simulink model "scattering_based_bi_teleop_pp_kalman"  (R2020b)
settings: Solver=FixedStepAuto  StartTime=0.0  StopTime=30  FixedStep=Ts  RelTol=1e-3
values from neighbouring files (symbols this model uses):
  A = 1    [four_channel_bilateral_teleoperation_kalman_params.m]    (also in four_channel_bilateral_teleoperation_params.m; kalman_test.m = [1 Ts Ts^2/2; 0 1 Ts; 0 0 1]; recursive_estimation.m = [1 Ts Ts^2/2; 0 1 Ts; 0 0 1]; scattering_based_bi_teleop_pf_kalman_params.m)
  b = 1    [scattering_based_bi_teleop_pf_kalman_params.m]    (also in scattering_based_bi_teleop_pf_params.m; scattering_based_bi_teleop_pp_kalman_params.m; scattering_based_bi_teleop_pp_params.m; scattering_based_bilateral_teleoperation_pp_params.m = 0.234)
  Be = 100    [four_channel_bilateral_teleoperation_architecture_params.m]    (also in four_channel_bilateral_teleoperation_kalman_params.m = 0; four_channel_bilateral_teleoperation_params.m = 0; scattering_based_bi_teleop_pf_kalman_params.m = 10; scattering_based_bi_teleop_pf_params.m = 10)
  Bh = 70    [four_channel_bilateral_teleoperation_architecture_params.m]    (also in four_channel_bilateral_teleoperation_kalman_params.m; four_channel_bilateral_teleoperation_params.m = 1.5; scattering_based_bi_teleop_pf_kalman_params.m = 1.5; scattering_based_bi_teleop_pf_params.m = 1.5)
  Bm = 1    [four_channel_bilateral_teleoperation_architecture_params.m]    (also in four_channel_bilateral_teleoperation_kalman_params.m = 0.8; four_channel_bilateral_teleoperation_params.m = 0.8; scattering_based_bi_teleop_pf_kalman_params.m = 0; scattering_based_bi_teleop_pf_params.m = 0)
  Bs = 1    [four_channel_bilateral_teleoperation_architecture_params.m]    (also in four_channel_bilateral_teleoperation_kalman_params.m = 3.2; four_channel_bilateral_teleoperation_params.m = 3.2; scattering_based_bi_teleop_pf_kalman_params.m = 40; scattering_based_bi_teleop_pf_params.m = 80)
  delay = 10    [scattering_based_bi_teleop_pf_kalman_params.m]    (also in scattering_based_bi_teleop_pf_params.m; scattering_based_bi_teleop_pp_kalman_params.m = 2; scattering_based_bi_teleop_pp_params.m; tank_based_bi_teleop_pf_kalman.m = 1)
  Dm = 5    [four_channel_bilateral_teleoperation_architecture_params.m]    (also in four_channel_bilateral_teleoperation_kalman_params.m = 0; four_channel_bilateral_teleoperation_params.m = 0; scattering_based_bi_teleop_pf_kalman_params.m = 0; scattering_based_bi_teleop_pf_params.m = 0)
  Ds = 10    [four_channel_bilateral_teleoperation_architecture_params.m]    (also in four_channel_bilateral_teleoperation_kalman_params.m = 0; four_channel_bilateral_teleoperation_params.m = 0; scattering_based_bi_teleop_pf_kalman_params.m = 0; scattering_based_bi_teleop_pf_params.m = 0)
  Fc = 1    [four_channel_bilateral_teleoperation_kalman_params.m]    (also in four_channel_bilateral_teleoperation_params.m = 0.5; scattering_based_bi_teleop_pf_kalman_params.m = 0.1; scattering_based_bi_teleop_pf_params.m = 0.1; scattering_based_bi_teleop_pp_kalman_params.m = 0.1)
  Filter = 8    [scattering_based_bi_teleop_pf_kalman_params.m]    (also in scattering_based_bi_teleop_pf_params.m = 10; scattering_based_bi_teleop_pp_kalman_params.m = 10; scattering_based_bi_teleop_pp_params.m = 10; tank_based_bi_teleop_pf_kalman.m = 100)
  Fip = 1    [four_channel_bilateral_teleoperation_kalman_params.m]    (also in four_channel_bilateral_teleoperation_params.m; scattering_based_bi_teleop_pf_kalman_params.m = 5; scattering_based_bi_teleop_pf_params.m = 5; scattering_based_bi_teleop_pp_kalman_params.m = 5)
  Ih = 2    [scattering_based_bi_teleop_pf_kalman_params.m]    (also in scattering_based_bi_teleop_pf_params.m; scattering_based_bi_teleop_pp_kalman_params.m; scattering_based_bi_teleop_pp_params.m; tank_based_bi_teleop_pf_kalman.m)
  Je = 0    [four_channel_bilateral_teleoperation_architecture_params.m]    (also in four_channel_bilateral_teleoperation_kalman_params.m; four_channel_bilateral_teleoperation_params.m; scattering_based_bi_teleop_pf_kalman_params.m; scattering_based_bi_teleop_pf_params.m)
  Jh = 0.5    [four_channel_bilateral_teleoperation_architecture_params.m]    (also in four_channel_bilateral_teleoperation_kalman_params.m; four_channel_bilateral_teleoperation_params.m = 0; scattering_based_bi_teleop_pf_kalman_params.m = 0; scattering_based_bi_teleop_pf_params.m = 0)
  Ke = 200    [four_channel_bilateral_teleoperation_architecture_params.m]    (also in four_channel_bilateral_teleoperation_kalman_params.m = 50; four_channel_bilateral_teleoperation_params.m; scattering_based_bi_teleop_pf_kalman_params.m; scattering_based_bi_teleop_pf_params.m)
  Kh = 2000    [four_channel_bilateral_teleoperation_architecture_params.m]    (also in four_channel_bilateral_teleoperation_kalman_params.m; four_channel_bilateral_teleoperation_params.m = 1; scattering_based_bi_teleop_pf_kalman_params.m = 1; scattering_based_bi_teleop_pf_params.m = 1)
  Km = 1    [four_channel_bilateral_teleoperation_architecture_params.m]    (also in four_channel_bilateral_teleoperation_kalman_params.m; four_channel_bilateral_teleoperation_params.m; scattering_based_bi_teleop_pf_kalman_params.m = 0; scattering_based_bi_teleop_pf_params.m = 0)
  Ks = 1    [four_channel_bilateral_teleoperation_architecture_params.m]    (also in four_channel_bilateral_teleoperation_kalman_params.m = 4; four_channel_bilateral_teleoperation_params.m = 4; scattering_based_bi_teleop_pf_kalman_params.m = 50; scattering_based_bi_teleop_pf_params.m = 100)
  Mm = 0.5    [four_channel_bilateral_teleoperation_architecture_params.m]    (also in four_channel_bilateral_teleoperation_kalman_params.m; four_channel_bilateral_teleoperation_params.m; scattering_based_bi_teleop_pf_kalman_params.m; scattering_based_bi_teleop_pf_params.m)
  Ms = 2    [four_channel_bilateral_teleoperation_architecture_params.m]    (also in four_channel_bilateral_teleoperation_kalman_params.m; four_channel_bilateral_teleoperation_params.m; scattering_based_bi_teleop_pf_kalman_params.m; scattering_based_bi_teleop_pf_params.m)
  Ph = 2000    [four_channel_bilateral_teleoperation_kalman_params.m]    (also in four_channel_bilateral_teleoperation_params.m = 50; scattering_based_bi_teleop_pf_kalman_params.m = 5; scattering_based_bi_teleop_pf_params.m = 5; scattering_based_bi_teleop_pp_kalman_params.m = 6)
  Ts = 0.001    [four_channel_bilateral_teleoperation_kalman_params.m]    (also in four_channel_bilateral_teleoperation_params.m; kalman_test.m; recursive_estimation.m; scattering_based_bi_teleop_pf_kalman_params.m)
  VarianceForces = 0.01    [four_channel_bilateral_teleoperation_kalman_params.m]    (also in four_channel_bilateral_teleoperation_params.m = 0; scattering_based_bi_teleop_pf_kalman_params.m; scattering_based_bi_teleop_pp_kalman_params.m; scattering_based_bi_teleop_pp_params.m)
  VarianceVelocities = 0.001    [four_channel_bilateral_teleoperation_kalman_params.m]    (also in four_channel_bilateral_teleoperation_params.m = 0; scattering_based_bi_teleop_pf_kalman_params.m = 1e-05; scattering_based_bi_teleop_pp_kalman_params.m = 1e-05; scattering_based_bi_teleop_pp_params.m = 1e-05)
undefined symbols (not defined in the file or in its folder): DiscIntNeverNeededParam
settings Model: Creator=anuj  LastModifiedBy=filippo

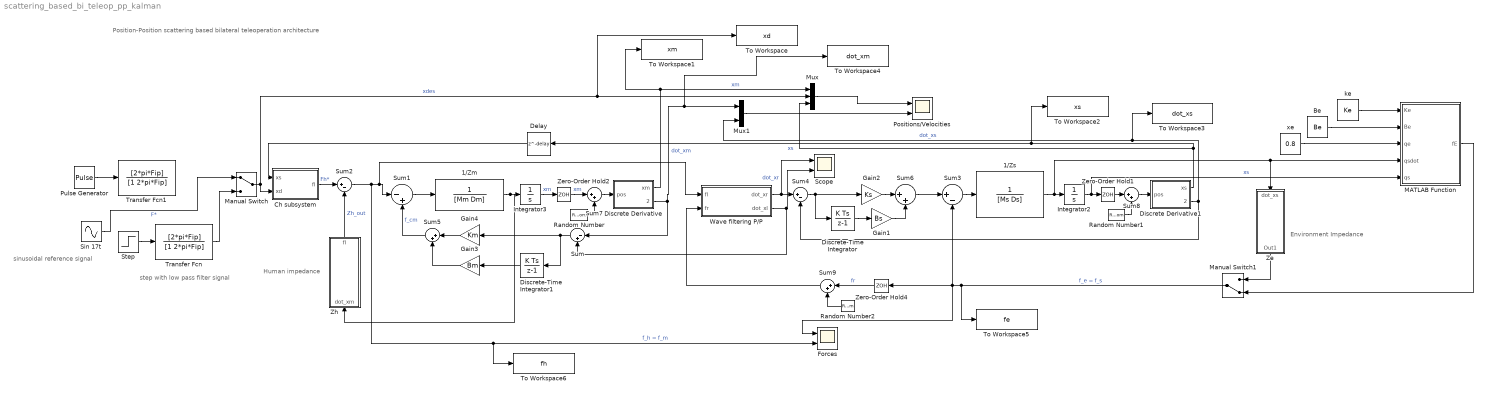
== system scattering_based_bi_teleop_pp_kalman ==
  note: Position-Position scattering based bilateral teleoperation architecture
  note: Environment Impedance
  note: Human impedance
  note: sinusoidal reference signal
  note: step with low pass filter signal
  1/Zm : TransferFcn  Denominator=[Mm Dm]
  1/Zs : TransferFcn  Denominator=[Ms Ds]
  Be : Constant  Value=Be
  Ch subsystem : Subsystem
  Delay : Delay  DelayLength=delay  SampleTime=Ts
  Discrete Derivative : Subsystem
  Discrete Derivative1 : Subsystem
  Discrete-Time Integrator : DiscreteIntegrator  SampleTime=-1  ICPrevOutput=DiscIntNeverNeededParam  ICPrevScaledInput=DiscIntNeverNeededParam
  Discrete-Time Integrator1 : DiscreteIntegrator  SampleTime=-1  ICPrevOutput=DiscIntNeverNeededParam  ICPrevScaledInput=DiscIntNeverNeededParam
  Forces : Scope  NumInputPorts=2
  Gain1 : Gain  Gain=Bs
  Gain2 : Gain  Gain=Ks
  Gain3 : Gain  Gain=Bm
  Gain4 : Gain  Gain=Km
  Integrator2 : Integrator
  Integrator3 : Integrator
  MATLAB Function : MATLAB Function  TreatAsAtomicUnit=on
  Manual Switch : ManualSwitch
  Manual Switch1 : ManualSwitch  CurrentSetting=0
  Mux : Mux  Inputs=3
  Mux1 : Mux  Inputs=2
  Positions/Velocities : Scope  NumInputPorts=2
  Pulse Generator : DiscretePulseGenerator  PulseType=Time based  Amplitude=A  PulseWidth=50  PhaseDelay=1
  Random Number : RandomNumber  Variance=VarianceVelocities  SampleTime=Ts
  Random Number1 : RandomNumber  Variance=VarianceVelocities  SampleTime=Ts
  Random Number2 : RandomNumber  Variance=VarianceForces  SampleTime=Ts
  Scope : Scope  NumInputPorts=2
  Sin 17t : Sin  Amplitude=A  Frequency=2*pi*Fc  SampleTime=0
  Step : Step  After=A  SampleTime=0
  Sum : Sum  Inputs=|-+
  Sum1 : Sum  Inputs=|-+
  Sum2 : Sum  Inputs=|+-
  Sum3 : Sum  Inputs=|+-
  Sum4 : Sum  Inputs=|+-
  Sum{5..9} (5 alike) : Sum  Inputs=|++
  To Workspace : ToWorkspace  VariableName=xd  SaveFormat=Timeseries  SampleTime=-1
  To Workspace1 : ToWorkspace  VariableName=xm  SaveFormat=Timeseries  SampleTime=-1
  To Workspace2 : ToWorkspace  VariableName=xs  SaveFormat=Timeseries  SampleTime=-1
  To Workspace3 : ToWorkspace  VariableName=dot_xs  SaveFormat=Timeseries  SampleTime=-1
  To Workspace4 : ToWorkspace  VariableName=dot_xm  SaveFormat=Timeseries  SampleTime=-1
  To Workspace5 : ToWorkspace  VariableName=fe  SaveFormat=Timeseries  SampleTime=-1
  To Workspace6 : ToWorkspace  VariableName=fh  SaveFormat=Timeseries  SampleTime=-1
  Transfer Fcn : TransferFcn  Numerator=[2*pi*Fip]  Denominator=[1 2*pi*Fip]
  Transfer Fcn1 : TransferFcn  Numerator=[2*pi*Fip]  Denominator=[1 2*pi*Fip]
  Wave filtering P/P : Subsystem
  Ze : Subsystem
  Zero-Order Hold1 : ZeroOrderHold  SampleTime=Ts
  Zero-Order Hold2 : ZeroOrderHold  SampleTime=Ts
  Zero-Order Hold4 : ZeroOrderHold  SampleTime=Ts
  Zh : Subsystem
  ke : Constant  Value=Ke
  xe : Constant  Value=0.8
  wires:
  Sum2/1 -> To Workspace6/1, Forces/2, Wave filtering P/P/1(fl), Sum1/1  "f_h = f_m"
  1/Zm/1 -> Zh/1(dot_xm), Integrator3/1
  Sum1/1 -> 1/Zm/1
  Sum3/1 -> 1/Zs/1
  Manual Switch1/1 -> To Workspace5/1, Forces/1, Zero-Order Hold4/1, Sum3/2  "f_e = f_s"
  Be/1 -> MATLAB Function/2(Be)
  xe/1 -> MATLAB Function/3(qe)
  ke/1 -> MATLAB Function/1(Ke)
  Transfer Fcn/1 -> Manual Switch/2
  Step/1 -> Transfer Fcn/1
  Zh/1(fl) -> Sum2/2  "Zh_out"
  Discrete Derivative1/2(dot_xs) -> To Workspace3/1, Mux1/2, Sum4/2  "dot_xs"
  1/Zs/1 -> Integrator2/1, Ze/1(dot_xs), MATLAB Function/4(qsdot)
  Integrator2/1 -> Zero-Order Hold1/1, MATLAB Function/5(qs)  "xs"
  Integrator3/1 -> Zero-Order Hold2/1  "xm"
  Discrete Derivative/2(dot_xm) -> To Workspace4/1, Mux1/1, Sum/1  "dot_xm"
  Ze/1(Out1) -> Manual Switch1/1
  MATLAB Function/1(fE) -> Manual Switch1/2
  Mux1/1 -> Positions/Velocities/2
  Mux/1 -> Positions/Velocities/1
  Manual Switch/1 -> To Workspace/1, Mux/2, Ch subsystem/2(xd)  "xdes"
  Ch subsystem/1(fl) -> Sum2/1  "Fh*"
  Sum6/1 -> Sum3/1
  Gain1/1 -> Sum6/2
  Gain2/1 -> Sum6/1
  Discrete-Time Integrator/1 -> Gain1/1
  Wave filtering P/P/1(dot_xr) -> Scope/1, Sum4/1  "dot_xr"
  Sum4/1 -> Discrete-Time Integrator/1, Gain2/1
  Gain4/1 -> Sum5/1
  Sum5/1 -> Sum1/2  "f_cm"
  Gain3/1 -> Sum5/2
  Pulse Generator/1 -> Transfer Fcn1/1
  Delay/1 -> Ch subsystem/1(xs)
  Sum/1 -> Gain4/1, Discrete-Time Integrator1/1
  Discrete-Time Integrator1/1 -> Gain3/1
  Wave filtering P/P/2(dot_xl) -> Sum/2, Scope/2
  Discrete Derivative/1(xm) -> Mux/1, To Workspace1/1  "xm"
  Zero-Order Hold2/1 -> Sum7/1  "xm"
  Random Number/1 -> Sum7/2
  Sum7/1 -> Discrete Derivative/1(pos)
  Zero-Order Hold1/1 -> Sum8/1
  Sum8/1 -> Discrete Derivative1/1(pos)
  Random Number1/1 -> Sum8/2
  Discrete Derivative1/1(xs) -> To Workspace2/1, Delay/1, Mux/3  "xs"
  Random Number2/1 -> Sum9/2
  Zero-Order Hold4/1 -> Sum9/1  "fr"
  Sum9/1 -> Wave filtering P/P/2(fr)
  Sin 17t/1 -> Manual Switch/1  "F*"

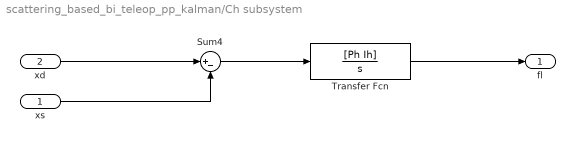
== system scattering_based_bi_teleop_pp_kalman/Ch subsystem ==
  xs : Inport
  xd : Inport  Port=2
  Sum4 : Sum  Inputs=|+-
  Transfer Fcn : TransferFcn  Numerator=[Ph Ih]  Denominator=[1 0]
  fl : Outport
  wires:
  xs/1 -> Sum4/2
  Sum4/1 -> Transfer Fcn/1
  xd/1 -> Sum4/1
  Transfer Fcn/1 -> fl/1

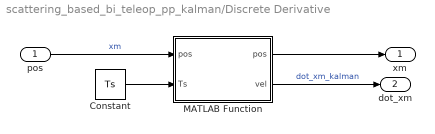
== system scattering_based_bi_teleop_pp_kalman/Discrete Derivative ==
  pos : Inport
  Constant : Constant  Value=Ts
  MATLAB Function : MATLAB Function  TreatAsAtomicUnit=on
  xm : Outport
  dot_xm : Outport  Port=2
  wires:
  pos/1 -> MATLAB Function/1("pos ")  "xm"
  Constant/1 -> MATLAB Function/2(Ts)
  MATLAB Function/1(pos) -> xm/1
  MATLAB Function/2(vel) -> dot_xm/1  "dot_xm_kalman"

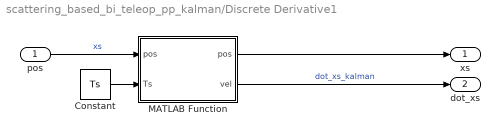
== system scattering_based_bi_teleop_pp_kalman/Discrete Derivative1 ==
  pos : Inport
  Constant : Constant  Value=Ts
  MATLAB Function : MATLAB Function  TreatAsAtomicUnit=on
  xs : Outport
  dot_xs : Outport  Port=2
  wires:
  pos/1 -> MATLAB Function/1("pos ")  "xs"
  Constant/1 -> MATLAB Function/2(Ts)
  MATLAB Function/1(pos) -> xs/1
  MATLAB Function/2(vel) -> dot_xs/1  "dot_xs_kalman"

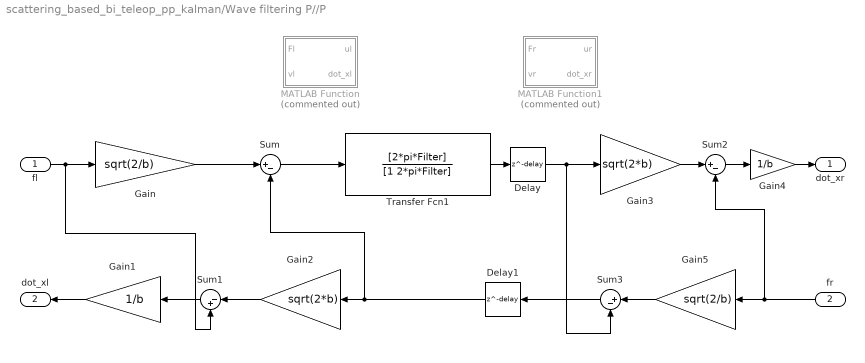
== system scattering_based_bi_teleop_pp_kalman/Wave filtering P//P ==
  fl : Inport
  fr : Inport  Port=2
  Delay : Delay  DelayLength=delay  SampleTime=Ts
  Delay1 : Delay  DelayLength=delay  SampleTime=Ts
  Gain : Gain  Gain=sqrt(2/b)
  Gain1 : Gain  Gain=1/b
  Gain2 : Gain  Gain=sqrt(2*b)
  Gain3 : Gain  Gain=sqrt(2*b)
  Gain4 : Gain  Gain=1/b
  Gain5 : Gain  Gain=sqrt(2/b)
  MATLAB Function : MATLAB Function  Commented=on  TreatAsAtomicUnit=on
  MATLAB Function1 : MATLAB Function  Commented=on  TreatAsAtomicUnit=on
  Sum : Sum  Inputs=|+-
  Sum1 : Sum  Inputs=|-+
  Sum2 : Sum  Inputs=|+-
  Sum3 : Sum  Inputs=|+-
  Transfer Fcn1 : TransferFcn  Numerator=[2*pi*Filter]  Denominator=[1 2*pi*Filter]
  dot_xr : Outport
  dot_xl : Outport  Port=2
  wires:
  Sum2/1 -> Gain4/1
  fl/1 -> Gain/1, Sum1/2
  Gain2/1 -> Sum1/1
  Gain3/1 -> Sum2/1
  Delay/1 -> Gain3/1, Sum3/2
  Sum1/1 -> Gain1/1
  Delay1/1 -> Sum/2, Gain2/1
  Transfer Fcn1/1 -> Delay/1
  Gain4/1 -> dot_xr/1
  Gain1/1 -> dot_xl/1
  fr/1 -> Gain5/1, Sum2/2
  Sum3/1 -> Delay1/1
  Sum/1 -> Transfer Fcn1/1
  Gain/1 -> Sum/1
  Gain5/1 -> Sum3/1

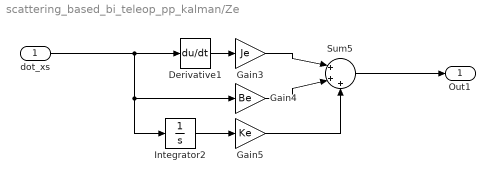
== system scattering_based_bi_teleop_pp_kalman/Ze ==
  dot_xs : Inport
  Derivative1 : Derivative
  Gain3 : Gain  Gain=Je
  Gain4 : Gain  Gain=Be
  Gain5 : Gain  Gain=Ke
  Integrator2 : Integrator
  Sum5 : Sum  Inputs=|+++
  Out1 : Outport
  wires:
  Gain4/1 -> Sum5/2
  Gain3/1 -> Sum5/1
  Gain5/1 -> Sum5/3
  Sum5/1 -> Out1/1
  Integrator2/1 -> Gain5/1
  dot_xs/1 -> Integrator2/1, Gain4/1, Derivative1/1
  Derivative1/1 -> Gain3/1

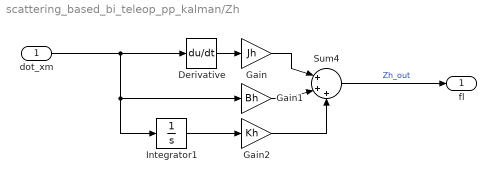
== system scattering_based_bi_teleop_pp_kalman/Zh ==
  dot_xm : Inport
  Derivative : Derivative
  Gain : Gain  Gain=Jh
  Gain1 : Gain  Gain=Bh
  Gain2 : Gain  Gain=Kh
  Integrator1 : Integrator
  Sum4 : Sum  Inputs=|+++
  fl : Outport
  wires:
  Derivative/1 -> Gain/1
  Integrator1/1 -> Gain2/1
  Gain2/1 -> Sum4/3
  Gain1/1 -> Sum4/2
  Gain/1 -> Sum4/1
  Sum4/1 -> fl/1  "Zh_out"
  dot_xm/1 -> Gain1/1, Integrator1/1, Derivative/1

== matlab function scattering_based_bi_teleop_pp_kalman/Wave filtering P//P/MATLAB Function ==
  data: Fl input; ul output; vl input; dot_xl output
function [ul, dot_xl] = left(Fl, vl)
    ul = sqrt(2/1)*Fl - vl;
    dot_xl = 1/1*(Fl-sqrt(2*1)*vl);
end

== matlab function scattering_based_bi_teleop_pp_kalman/MATLAB Function ==
  data: Ke input; fE output; Be input; qe input; qsdot input; qs input
function fE = environment(Ke, Be, qe, qsdot, qs)
    if qs > qe
        fE = Ke * (qs - qe) + Be * qsdot; % Plot both contributions Ke and Be
    else
        fE = 0;
    end
end

== matlab function scattering_based_bi_teleop_pp_kalman/Wave filtering P//P/MATLAB Function1 ==
  data: Fr input; ur output; vr input; dot_xr output
function [ur, dot_xr] = right(Fr, vr)
    ur = sqrt(2/1)*Fr - vr;
    dot_xr = -1/1*(Fr-sqrt(2*1)*vr);
end

== matlab function scattering_based_bi_teleop_pp_kalman/Discrete Derivative/MATLAB Function ==
  data: pos output; pos input; vel output; Ts input
function [pos, vel] = kalman(pos, Ts)
    persistent P A C Q R x_filter_old P_filter_old
    if isempty(P)
        P = 0;
        x_filter_old=[pos; 0];
        P_filter_old=0.1*eye(2);
        A=[1 Ts; 0 1];
        C=[1 0];
        q=1000000;
        Q=q*[Ts^2/2;Ts]*[Ts^2/2;Ts]';
        R=1;
    end

    % Prediction step (A priori estimation)
    x_kplus1_k = A*x_filter_old;
    P_kplus1_k = A*P_filter_old*A'+Q;

    % Compute the kalman gain
    K = P_kplus1_k * C' * inv(C * P_kplus1_k * C' + R);

    % Calculate the estimation step
    x_kplus1_kplus1 = x_kplus1_k + K *(pos - C * x_kplus1_k);
    P_kplus1_kplus1 = P_kplus1_k - P_kplus1_k * C' * inv(C * P_kplus1_k * C' + R) * C * P_kplus1_k;
    
    % Next step iteration
    x_filter_old = x_kplus1_kplus1;
    P_filter_old = P_kplus1_kplus1;
    
    pos = x_kplus1_kplus1(1,:);
    vel = x_kplus1_kplus1(2,:);
end

== matlab function scattering_based_bi_teleop_pp_kalman/Discrete Derivative1/MATLAB Function ==
  data: pos output; pos input; vel output; Ts input
function [pos, vel] = kalman(pos, Ts)
    persistent P A C Q R x_filter_old P_filter_old
    if isempty(P)
        P = 0;
        x_filter_old=[pos; 0];
        P_filter_old=0.1*eye(2);
        A=[1 Ts; 0 1];
        C=[1 0];
        q=1000000;
        Q=q*[Ts^2/2;Ts]*[Ts^2/2;Ts]';
        R=1;
    end

    % Prediction step (A priori estimation)
    x_kplus1_k = A*x_filter_old;
    P_kplus1_k = A*P_filter_old*A'+Q;

    % Compute the kalman gain
    K = P_kplus1_k * C' * inv(C * P_kplus1_k * C' + R);

    % Calculate the estimation step
    x_kplus1_kplus1 = x_kplus1_k + K *(pos - C * x_kplus1_k);
    P_kplus1_kplus1 = P_kplus1_k - P_kplus1_k * C' * inv(C * P_kplus1_k * C' + R) * C * P_kplus1_k;
    
    % Next step iteration
    x_filter_old = x_kplus1_kplus1;
    P_filter_old = P_kplus1_kplus1;
    
    pos = x_kplus1_kplus1(1,:);
    vel = x_kplus1_kplus1(2,:);
end
